simulink model "lab3"  (R2014a)
settings: Solver=ode15s  StartTime=0.0  StopTime=1  RelTol=1e-3
undefined symbols (not defined in the file): D1, Delta
libraries: powerlib x22
settings Model: Creator=Thodoris  LastModifiedBy=Thodoris

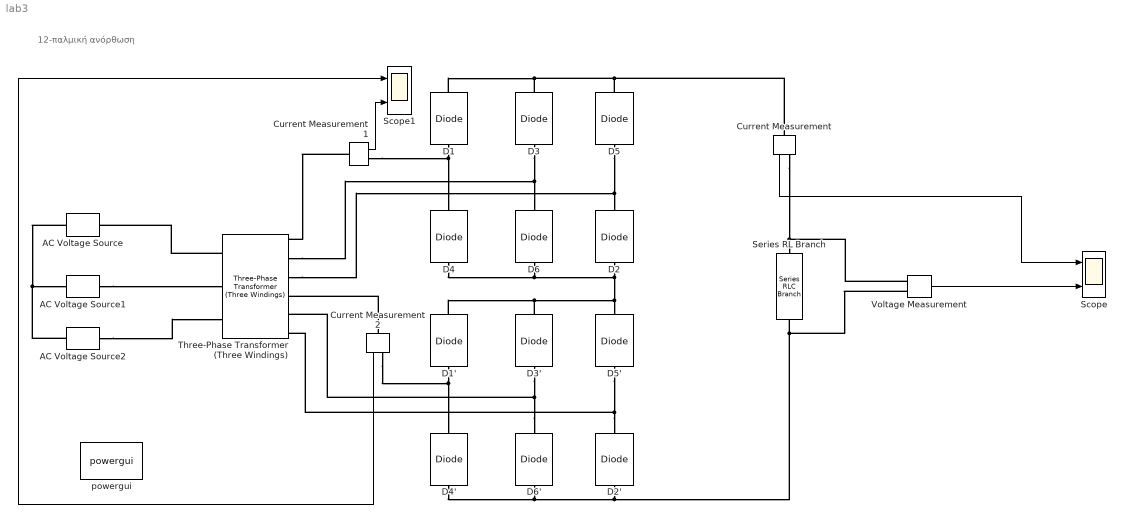
== system lab3 ==
  note: 12-παλμική ανόρθωση
  AC Voltage Source : powerlib/Electrical Sources/AC Voltage Source  Amplitude=380  Phase=0  Frequency=50  SampleTime=0  Measurements=None
  AC Voltage Source1 : powerlib/Electrical Sources/AC Voltage Source  Amplitude=380  Phase=-120  Frequency=50  SampleTime=0  Measurements=None
  AC Voltage Source2 : powerlib/Electrical Sources/AC Voltage Source  Amplitude=380  Phase=120  Frequency=50  SampleTime=0  Measurements=None
  Current Measurement2 : powerlib/Measurements/Current Measurement  PhasorSimulation=off  OutputType=Complex  PSBequivalent=0
  Current Measurement : powerlib/Measurements/Current Measurement  PhasorSimulation=off  OutputType=Complex  PSBequivalent=0
  Current Measurement1 : powerlib/Measurements/Current Measurement  PhasorSimulation=off  OutputType=Complex  PSBequivalent=0
  D{1..6} (6 alike) : powerlib/Power Electronics/Diode  Ron=0.001  Lon=0  Vf=0.8  IC=0  UseSnubber=off  Rs=500  Cs=250e-9  Measurements=off
  D1' : powerlib/Power Electronics/Diode  Ron=0.001  Lon=0  Vf=0.8  IC=0  UseSnubber=off  Rs=500  Cs=250e-9  Measurements=off
  D2' : powerlib/Power Electronics/Diode  Ron=0.001  Lon=0  Vf=0.8  IC=0  UseSnubber=off  Rs=500  Cs=250e-9  Measurements=off
  D3' : powerlib/Power Electronics/Diode  Ron=0.001  Lon=0  Vf=0.8  IC=0  UseSnubber=off  Rs=500  Cs=250e-9  Measurements=off
  D4' : powerlib/Power Electronics/Diode  Ron=0.001  Lon=0  Vf=0.8  IC=0  UseSnubber=off  Rs=500  Cs=250e-9  Measurements=off
  D5' : powerlib/Power Electronics/Diode  Ron=0.001  Lon=0  Vf=0.8  IC=0  UseSnubber=off  Rs=500  Cs=250e-9  Measurements=off
  D6' : powerlib/Power Electronics/Diode  Ron=0.001  Lon=0  Vf=0.8  IC=0  UseSnubber=off  Rs=500  Cs=250e-9  Measurements=off
  Scope : Scope  NumInputPorts=2
      settings: YMin=0~0  YMax=50~400
  Scope1 : Scope  NumInputPorts=2
      settings: YMin=0~-5  YMax=400~5
  Series RL Branch : powerlib/Elements/Series RLC Branch  LConnTagsString=__new0  RConnTagsString=__new0  BranchType=RL  Resistance=10  Inductance=650e-3  SetiL0=off  InitialCurrent=0  Capacitance=1e-6  Setx0=off  InitialVoltage=0  Measurements=None
  Three-Phase Transformer (Three Windings) : powerlib/Elements/Three-Phase Transformer (Three Windings)  Winding1Connection=Y  UNITS=pu  NominalPower=[ 250e6 , 50 ]  Winding1=[ 380 , 0.002 , 0.08 ]  Winding2Connection=Y  Winding2=[ 100 , 0.002 , 0.08 ]  Winding3Connection=Delta (D1)  Winding3=[ 100 , 0.002 , 0.08 ]  SetSaturation=off  Rm=500  Lm=500  Saturation=[ 0,0 ; 0.0024,1.2 ; 1.0,1.52 ]  Hysteresis=off  DataFile='hysteresis'  SetInitialFlux=off  InitialFluxes=[0.8 -0.8 0.7]  Measurements=None  MoreParameters=off  BreakLoop=off  DataType=off  TransfoNumber=1
  Voltage Measurement : powerlib/Measurements/Voltage Measurement  PhasorSimulation=off  OutputType=Complex  PSBequivalent=0
  powergui : powerlib/powergui  Priority=1  SimulationMode=Continuous  SolverType=Tustin  SampleTime=50e-6  frequency=60  SPID=off  DisableSnubberDevices=off  DisableRonSwitches=off  DisableVfSwitches=off  SwTol=0  Interpol=off  DisplayEquations=off  Ts=0  methode=off  frequencyindice=50  Pbase=100e6  ErrMax=1e-4  Iterations=50  UnitsV=kV  UnitsW=MW  FunctionMessages=off  echomessages=off  HookPort=off  EnableUseOfTLC=off  x0status=blocks  RestoreLinks=warning  ResistiveCurrentMeasurement=off  Frange=[0:2:500]  Ylog=off  Xlog=on  ShowGrid=off  save=off  variable=ZData  structure=0  ZoomFFT=off  StartTime=0.0  cycles=1  DisplayStyle=1  fundamental=60  FreqAxis=off  MaxFrequency=1000  frequencyindicesteady=1  RmsSteady=1  display=off
  wires:
  Voltage Measurement/1 -> Scope/2
  Current Measurement/1 -> Scope/1
  Current Measurement1/1 -> Scope1/2
  Current Measurement2/1 -> Scope1/1
  connections:
  AC Voltage Source/LConn1 -- AC Voltage Source2/LConn1 -- AC Voltage Source1/LConn1
  AC Voltage Source1/RConn1 -- Three-Phase Transformer (Three Windings)/LConn2
  AC Voltage Source2/RConn1 -- Three-Phase Transformer (Three Windings)/LConn3
  D5/LConn1 -- Three-Phase Transformer (Three Windings)/RConn3 -- D2/RConn1
  D3/LConn1 -- Three-Phase Transformer (Three Windings)/RConn2 -- D6/RConn1
  D1/LConn1 -- Current Measurement1/RConn1 -- D4/RConn1
  D2'/RConn1 -- D5'/LConn1 -- Three-Phase Transformer (Three Windings)/RConn6
  D6'/RConn1 -- D3'/LConn1 -- Three-Phase Transformer (Three Windings)/RConn5
  D1'/LConn1 -- Current Measurement2/RConn1 -- D4'/RConn1
  D2/LConn1 -- D6/LConn1 -- D4/LConn1 -- D3'/RConn1 -- D1'/RConn1 -- D5'/RConn1
  D4'/LConn1 -- D6'/LConn1 -- D2'/LConn1 -- Voltage Measurement/LConn2 -- Series RL Branch/RConn1
  D1/RConn1 -- Current Measurement/LConn1 -- D5/RConn1 -- D3/RConn1
  Voltage Measurement/LConn1 -- Current Measurement/RConn1 -- Series RL Branch/LConn1
  Current Measurement1/LConn1 -- Three-Phase Transformer (Three Windings)/RConn1
  Current Measurement2/LConn1 -- Three-Phase Transformer (Three Windings)/RConn4
  Three-Phase Transformer (Three Windings)/LConn1 -- AC Voltage Source/RConn1
